simulink model "sm_parts_all"  (R2019a)
settings: Solver=VariableStepAuto  StartTime=0.0  StopTime=10.0  RelTol=1e-3  EnableMultiTasking=on
undefined symbols (not defined in the file): X, Y, Z
libraries: sm_lib x19, Multibody_Parts_Lib x18, nesl_utility x1
Description:
  | Copyright 2017-2019 The MathWorks, Inc.
settings Model: Creator=smiller  LastModifiedBy=smiller
settings DataIOCC: LimitDataPoints=on  ReturnWorkspaceOutputs=off
settings OptimizationCC: LifeSpan=inf
settings DebuggingCC: AllowSymbolicDim=off  PregeneratedLibrarySubsystemCodeDiagnostic=none  SFUnexpectedBacktrackingDiag=warning  SFNoUnconditionalDefaultTransitionDiag=warning  SFExecutionAtInitializationDiag=none  ArithmeticOperatorsInVariantConditions=warning
settings SFSimCC: SimUseLocalCustomCode=off
settings RTWCC: RTWUseLocalCustomCode=off
settings CodeAppCC: StateflowObjectComments=on
settings GRTTargetCC: TargetLangStandard=C89/C90 (ANSI)  GeneratePreprocessorConditionals=Disable all
settings ConfigComp: CovMetricSettings=dw  CovHtmlReporting=on  CovSaveCumulativeToWorkspaceVar=on  CovSaveSingleToWorkspaceVar=on  CovExternalEMLEnable=off  CovSFcnEnable=off
settings SimscapeCC: SimscapeNormalizeSystem=off  SimscapeLogType=all  SimscapeLogDataHistory=10000
settings ConfigurationSet: Description=SimMechanics 2G
settings ExplorerConfigSet: InternalSimMechanicsExplorerSettings="<ExplorerConfiguration><canonicalview>default</canonicalview><AnimationSetting><BasePlaybackSpeed>1.0</BasePlaybackSpeed><PlaybackSpeedFactor>1.0</PlaybackSpeedFactor></AnimationSetting><TilePanel><TileInfo><Tiles Columns=\"1\" Count=\"1\" Rows=\"1\"><Column Left=\"2\" Weight=\"1\"/><Column Left=\"401\"/><Row Top=\"2\" Weight=\"1\"/><Row Top=\"205\"/><Tile Height=\"1\" Width=\"1\" X=\"0\" Y=\"0\"/></Tiles></TileInfo><SceneInfo><SceneViewer><BGColor><R>1</R><G>1</G><B>1</B></BGColor><Camera><DoPerspective>off</DoPerspective><Position><X>-0.71015375614700837</X><Y>0.14184611226395488</Y><Z>-0.013997968745046566</Z></Position><Center><X>0.28084060208517991</X><Y>0.025638016485088261</Y><Z>-0.080525109277487794</Z></Center><Up><X>0.11482264391220898</X><Y>0.99308884035982059</Y><Z>-0.024296411212304969</Z></Up><ViewLimDist>1</ViewLimDist><YLim>0.095367858286087334</YLim><XLim>0.19171889036893844</XLim></Camera></SceneViewer></SceneInfo></TilePanel><MechEditorPanel><Cameras/><GfxPanelCameraMap/><VideoCreator><PlaybackSpeedRatio>1.0</PlaybackSpeedRatio><FrameRate>30</FrameRate><VideoFormat>Motion JPEG AVI</VideoFormat><FrameSize>auto</FrameSize></VideoCreator></MechEditorPanel></ExplorerConfiguration>"

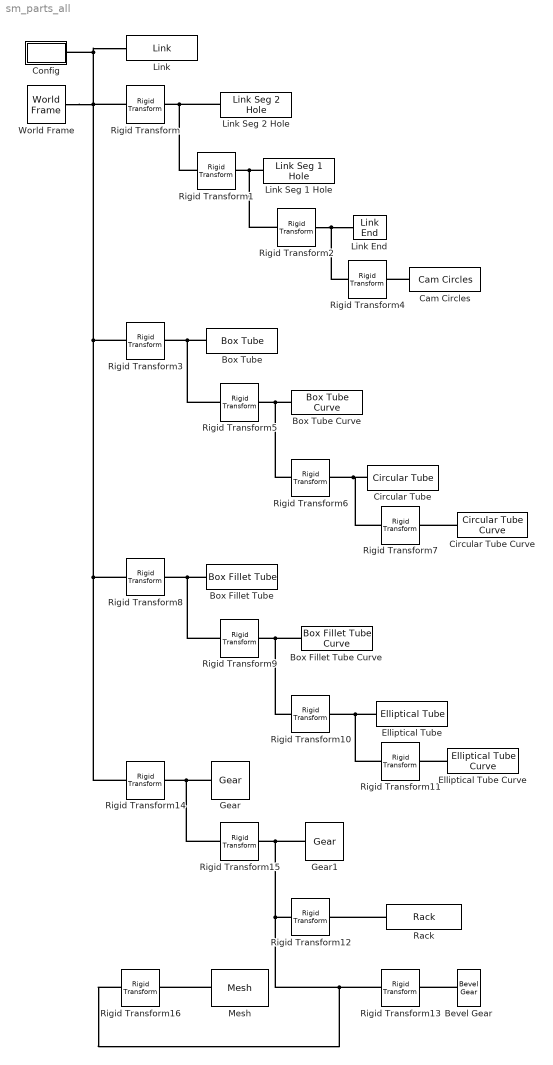
== system sm_parts_all ==
  Bevel Gear : Multibody_Parts_Lib/Gears/Bevel Gear  gear_ra=0.03  gear_th=0.01  gear_ca=90/2  gear_hr=0.002  gear_rho=7000  gear_clr=[0.0 0.4 0.6]  gear_opc=1  popup_markings=Two  mark_radius_range=[0.7 0.8]  mark_angle_range=60  mark_color=[1 1 1]
      settings: SourceProductName=Simscape Multibody Parts Library
  Box Fillet Tube : Multibody_Parts_Lib/Extrusions/Box Fillet Tube  box_ox=0.02  box_ix=0.01  box_oy=0.028  box_iy=0.018  rad_o=0.005  rad_i=0.002  box_len=0.05  box_rho=7000  box_color=[0 0.4 0.6]  box_opc=1
      settings: SourceProductName=Simscape Multibody Parts Library
  Box Fillet Tube Curve : Multibody_Parts_Lib/Extrusions/Box Fillet Tube Curve  box_ox=0.02  box_ix=0.01  box_oy=0.028  box_iy=0.018  rad_o=0.005  rad_i=0.002  arc_rad=0.05  arc_angle=45  popup_arcdir=Z  box_rho=7000  box_color=[0 0.4 0.6]  box_opc=1
      settings: SourceProductName=Simscape Multibody Parts Library
  Box Tube : Multibody_Parts_Lib/Extrusions/Box Tube  box_ox=0.02  box_ix=0.01  box_oy=0.028  box_iy=0.018  box_len=0.05  box_rho=7000  box_color=[0 0.4 0.6]  box_opc=1
      settings: SourceProductName=Simscape Multibody Parts Library
  Box Tube Curve : Multibody_Parts_Lib/Extrusions/Box Tube Curve  box_ox=0.02  box_ix=0.01  box_oy=0.028  box_iy=0.018  arc_rad=0.05  arc_angle=45  popup_arcdir=Z  box_rho=7000  box_color=[0 0.4 0.6]  box_opc=1
      settings: SourceProductName=Simscape Multibody Parts Library
  Cam Circles : Multibody_Parts_Lib/Linkages/Cam Circles  rad_b=0.02  rad_f=0.01  radhb=0.005  radhf=0.005  cam_len=0.05  cam_thickness=0.01  cam_rho=7000  cam_color=[0 0.4 0.6]  cam_opc=1
      settings: SourceProductName=Simscape Multibody Parts Library
  Circular Tube : Multibody_Parts_Lib/Extrusions/Circular Tube  circ_radout=0.015  circ_radin=0.01  deg_1=45  deg_2=315  circ_len=0.05  circ_rho=7000  circ_color=[0 0.4 0.6]  circ_opc=1
      settings: SourceProductName=Simscape Multibody Parts Library
  Circular Tube Curve : Multibody_Parts_Lib/Extrusions/Circular Tube Curve  circ_radout=0.015  circ_radin=0.01  deg_1=45  deg_2=315  arc_rad=0.05  arc_angle=45  popup_arcdir=Z  circ_rho=7000  circ_color=[0 0.4 0.6]  circ_opc=1
      settings: SourceProductName=Simscape Multibody Parts Library
  Config : Subsystem
  Elliptical Tube : Multibody_Parts_Lib/Extrusions/Elliptical Tube  rad_a=0.006  rad_b=0.015  deg_1=10  deg_2=350  ctr=0.7  ell_len=0.05  ell_rho=7000  ell_color=[0 0.4 0.6]  ell_opc=1
      settings: SourceProductName=Simscape Multibody Parts Library
  Elliptical Tube Curve : Multibody_Parts_Lib/Extrusions/Elliptical Tube Curve  rad_a=0.006  rad_b=0.015  deg_1=10  deg_2=350  ctr=0.7  arc_rad=0.05  arc_angle=45  popup_arcdir=Z  ell_rho=7000  ell_color=[0 0.4 0.6]  ell_opc=1
      settings: SourceProductName=Simscape Multibody Parts Library
  Gear : Multibody_Parts_Lib/Gears/Gear  popup_gear_type=External  gear_pd=0.035  gear_nt=12  gear_th=0.02  gear_rh=0.005  gear_rt=0.02  gear_rho=7000  gear_clr=[0.0 0.4 0.6]  gear_opc=1  popup_ad_dd=Default  gear_ad=0.125/12  gear_dd=1.157*0.125/12  popup_markings=Two  mark_radius_range=[0.6 0.7]  mark_angle_range=60  mark_color=[1 1 1]
      settings: SourceProductName=Simscape Multibody Parts Library
  Gear1 : Multibody_Parts_Lib/Gears/Gear  popup_gear_type=Internal  gear_pd=0.035  gear_nt=12  gear_th=0.02  gear_rh=0.005  gear_rt=0.002  gear_rho=7000  gear_clr=[0.0 0.4 0.6]  gear_opc=1  popup_ad_dd=Default  gear_ad=0.125/12  gear_dd=1.157*0.125/12  popup_markings=Two  mark_radius_range=[1.23 1.28]  mark_angle_range=60  mark_color=[1 1 1]
      settings: SourceProductName=Simscape Multibody Parts Library
  Link : Multibody_Parts_Lib/Linkages/Link  link_len=0.05  link_width=0.025  link_radh=0.005  link_numh=3  link_thickness=0.01  link_rho=7000  link_color=[0 0.4 0.6]  link_opc=1
      settings: SourceProductName=Simscape Multibody Parts Library
  Link End : Multibody_Parts_Lib/Linkages/Link End  circ_radout=0.025/2  circ_radin=0.005  popup_holelr=+X  deg_1=-90  deg_2=90  circ_len=0.01  circ_rho=7000  circ_color=[0 0.4 0.6]  circ_opc=1
      settings: SourceProductName=Simscape Multibody Parts Library
  Link Seg 1 Hole : Multibody_Parts_Lib/Linkages/Link Seg 1 Hole  link_len=0.05  link_width=0.025  link_radh=0.005  link_holelr=+X  link_thickness=0.01  link_rho=7000  link_color=[0 0.4 0.6]  link_opc=1
      settings: SourceProductName=Simscape Multibody Parts Library
  Link Seg 2 Hole : Multibody_Parts_Lib/Linkages/Link Seg 2 Hole  link_len=0.05  link_width=0.025  link_radh=0.005  link_thickness=0.01  link_rho=7000  link_color=[0 0.4 0.6]  link_opc=1
      settings: SourceProductName=Simscape Multibody Parts Library
  Mesh : Multibody_Parts_Lib/Basic/Mesh  mesh_lenx=0.06  mesh_leny=0.03  mesh_hx=0.0045  mesh_hy=0.0045  mesh_numhx=6  mesh_numhy=3  mesh_thickness=0.02  mesh_rho=7000  mesh_color=[0 0.4 0.6]  mesh_opc=1
      settings: SourceProductName=Simscape Multibody Parts Library
  Rack : Multibody_Parts_Lib/Gears/Rack  rack_tp=0.01  rack_nt=5  rack_tb=0.006  rack_th=0.006  rack_rho=7000  rack_clr=[0.5 0.5 0.5]  rack_opc=1  popup_ad_dd=Default  rack_ad=0.052/pi  rack_dd=1.157*0.052/pi
      settings: SourceProductName=Simscape Multibody Parts Library
  Rigid Transform{,1..2,4} (4 alike) : sm_lib/Frames and Transforms/Rigid Transform  TranslationMethod=StandardAxis  TranslationStandardOffset=0.05  TranslationLengthUnit=m  TranslationStandardAxis=+Y  TranslationCartesianOffset=[0 0 0]  TranslationROffset=0  TranslationROffsetUnits=m  TranslationZOffset=0  TranslationZOffsetUnits=m  TranslationThetaOffset=0  TranslationThetaOffsetUnits=deg  RotationMethod=None  RotationAngleUnits=deg  RotationStandardAxis=+Z  RotationAngle=0.0  RotationArbitraryAxis=[0 0 1]  FollAlignAxisA=+X  BaseAlignAxisA=+Y  FollAlignAxisB=+Y  BaseAlignAxisB=+Z  RotationSequenceAxes=FollowerAxes  RotationSequence=XYX  RotationSequenceAngles=[0 0 0]  RotationSequenceAnglesUnits=deg  RotationMatrix=[1 0 0; 0 1 0; 0 0 1]
  Rigid Transform{5..7,9..11,15} (7 alike) : sm_lib/Frames and Transforms/Rigid Transform  TranslationMethod=StandardAxis  TranslationStandardOffset=0.05  TranslationLengthUnit=m  TranslationStandardAxis=+Y  TranslationCartesianOffset=[0 0 0]  TranslationROffset=0  TranslationROffsetUnits=m  TranslationZOffset=0  TranslationZOffsetUnits=m  TranslationThetaOffset=0  TranslationThetaOffsetUnits=deg  RotationMethod=None  RotationAngleUnits=deg  RotationStandardAxis=+Y  RotationAngle=0  RotationArbitraryAxis=[0 0 1]  FollAlignAxisA=+X  BaseAlignAxisA=+Y  FollAlignAxisB=+Y  BaseAlignAxisB=+Z  RotationSequenceAxes=FollowerAxes  RotationSequence=XYX  RotationSequenceAngles=[0 0 0]  RotationSequenceAnglesUnits=deg  RotationMatrix=[1 0 0; 0 1 0; 0 0 1]
  Rigid Transform12 : sm_lib/Frames and Transforms/Rigid Transform  TranslationMethod=StandardAxis  TranslationStandardOffset=0.05  TranslationLengthUnit=m  TranslationStandardAxis=+Y  TranslationCartesianOffset=[0 0 0]  TranslationROffset=0  TranslationROffsetUnits=m  TranslationZOffset=0  TranslationZOffsetUnits=m  TranslationThetaOffset=0  TranslationThetaOffsetUnits=deg  RotationMethod=AlignedAxes  RotationAngleUnits=deg  RotationStandardAxis=+Y  RotationAngle=0  RotationArbitraryAxis=[0 0 1]  FollAlignAxisA=+Z  BaseAlignAxisA=+Y  FollAlignAxisB=+Y  BaseAlignAxisB=+X  RotationSequenceAxes=FollowerAxes  RotationSequence=XYX  RotationSequenceAngles=[0 0 0]  RotationSequenceAnglesUnits=deg  RotationMatrix=[1 0 0; 0 1 0; 0 0 1]
  Rigid Transform13 : sm_lib/Frames and Transforms/Rigid Transform  TranslationMethod=StandardAxis  TranslationStandardOffset=0.1  TranslationLengthUnit=m  TranslationStandardAxis=+Y  TranslationCartesianOffset=[0 0 0]  TranslationROffset=0  TranslationROffsetUnits=m  TranslationZOffset=0  TranslationZOffsetUnits=m  TranslationThetaOffset=0  TranslationThetaOffsetUnits=deg  RotationMethod=StandardAxis  RotationAngleUnits=deg  RotationStandardAxis=+X  RotationAngle=-75  RotationArbitraryAxis=[0 0 1]  FollAlignAxisA=+X  BaseAlignAxisA=+Y  FollAlignAxisB=+Y  BaseAlignAxisB=+Z  RotationSequenceAxes=FollowerAxes  RotationSequence=XYX  RotationSequenceAngles=[0 0 0]  RotationSequenceAnglesUnits=deg  RotationMatrix=[1 0 0; 0 1 0; 0 0 1]
  Rigid Transform14 : sm_lib/Frames and Transforms/Rigid Transform  TranslationMethod=StandardAxis  TranslationStandardOffset=0.15  TranslationLengthUnit=m  TranslationStandardAxis=-X  TranslationCartesianOffset=[0 0 0]  TranslationROffset=0  TranslationROffsetUnits=m  TranslationZOffset=0  TranslationZOffsetUnits=m  TranslationThetaOffset=0  TranslationThetaOffsetUnits=deg  RotationMethod=StandardAxis  RotationAngleUnits=deg  RotationStandardAxis=+Y  RotationAngle=0  RotationArbitraryAxis=[0 0 1]  FollAlignAxisA=+X  BaseAlignAxisA=+Y  FollAlignAxisB=+Y  BaseAlignAxisB=+Z  RotationSequenceAxes=FollowerAxes  RotationSequence=XYX  RotationSequenceAngles=[0 0 0]  RotationSequenceAnglesUnits=deg  RotationMatrix=[1 0 0; 0 1 0; 0 0 1]
  Rigid Transform16 : sm_lib/Frames and Transforms/Rigid Transform  TranslationMethod=StandardAxis  TranslationStandardOffset=0.15  TranslationLengthUnit=m  TranslationStandardAxis=+Y  TranslationCartesianOffset=[-0.2 0.05 0]  TranslationROffset=0  TranslationROffsetUnits=m  TranslationZOffset=0  TranslationZOffsetUnits=m  TranslationThetaOffset=0  TranslationThetaOffsetUnits=deg  RotationMethod=StandardAxis  RotationAngleUnits=deg  RotationStandardAxis=+Y  RotationAngle=0  RotationArbitraryAxis=[0 0 1]  FollAlignAxisA=+X  BaseAlignAxisA=+Y  FollAlignAxisB=+Y  BaseAlignAxisB=+Z  RotationSequenceAxes=FollowerAxes  RotationSequence=XYX  RotationSequenceAngles=[0 0 0]  RotationSequenceAnglesUnits=deg  RotationMatrix=[1 0 0; 0 1 0; 0 0 1]
  Rigid Transform3 : sm_lib/Frames and Transforms/Rigid Transform  TranslationMethod=StandardAxis  TranslationStandardOffset=0.05  TranslationLengthUnit=m  TranslationStandardAxis=-X  TranslationCartesianOffset=[0 0 0]  TranslationROffset=0  TranslationROffsetUnits=m  TranslationZOffset=0  TranslationZOffsetUnits=m  TranslationThetaOffset=0  TranslationThetaOffsetUnits=deg  RotationMethod=StandardAxis  RotationAngleUnits=deg  RotationStandardAxis=+Y  RotationAngle=80  RotationArbitraryAxis=[0 0 1]  FollAlignAxisA=+X  BaseAlignAxisA=+Y  FollAlignAxisB=+Y  BaseAlignAxisB=+Z  RotationSequenceAxes=FollowerAxes  RotationSequence=XYX  RotationSequenceAngles=[0 0 0]  RotationSequenceAnglesUnits=deg  RotationMatrix=[1 0 0; 0 1 0; 0 0 1]
  Rigid Transform8 : sm_lib/Frames and Transforms/Rigid Transform  TranslationMethod=StandardAxis  TranslationStandardOffset=0.1  TranslationLengthUnit=m  TranslationStandardAxis=-X  TranslationCartesianOffset=[0 0 0]  TranslationROffset=0  TranslationROffsetUnits=m  TranslationZOffset=0  TranslationZOffsetUnits=m  TranslationThetaOffset=0  TranslationThetaOffsetUnits=deg  RotationMethod=StandardAxis  RotationAngleUnits=deg  RotationStandardAxis=+Y  RotationAngle=80  RotationArbitraryAxis=[0 0 1]  FollAlignAxisA=+X  BaseAlignAxisA=+Y  FollAlignAxisB=+Y  BaseAlignAxisB=+Z  RotationSequenceAxes=FollowerAxes  RotationSequence=XYX  RotationSequenceAngles=[0 0 0]  RotationSequenceAnglesUnits=deg  RotationMatrix=[1 0 0; 0 1 0; 0 0 1]
  World Frame : sm_lib/Frames and Transforms/World Frame
  connections:
  World Frame/RConn1 -- Rigid Transform14/LConn1 -- Rigid Transform8/LConn1 -- Rigid Transform3/LConn1 -- Link/LConn1 -- Config/LConn1 -- Rigid Transform/LConn1
  Link Seg 2 Hole/LConn1 -- Rigid Transform1/LConn1 -- Rigid Transform/RConn1
  Link Seg 1 Hole/LConn1 -- Rigid Transform2/LConn1 -- Rigid Transform1/RConn1
  Rigid Transform2/RConn1 -- Rigid Transform4/LConn1 -- Link End/LConn1
  Box Tube/LConn1 -- Rigid Transform5/LConn1 -- Rigid Transform3/RConn1
  Cam Circles/LConn1 -- Rigid Transform4/RConn1
  Box Tube Curve/LConn1 -- Rigid Transform6/LConn1 -- Rigid Transform5/RConn1
  Circular Tube/LConn1 -- Rigid Transform7/LConn1 -- Rigid Transform6/RConn1
  Circular Tube Curve/LConn1 -- Rigid Transform7/RConn1
  Rigid Transform9/LConn1 -- Box Fillet Tube/LConn1 -- Rigid Transform8/RConn1
  Rigid Transform10/LConn1 -- Box Fillet Tube Curve/LConn1 -- Rigid Transform9/RConn1
  Rigid Transform11/LConn1 -- Elliptical Tube/LConn1 -- Rigid Transform10/RConn1
  Elliptical Tube Curve/LConn1 -- Rigid Transform11/RConn1
  Rigid Transform15/RConn1 -- Rigid Transform16/LConn1 -- Rigid Transform13/LConn1 -- Rigid Transform12/LConn1 -- Gear1/RConn1
  Rack/RConn1 -- Rigid Transform12/RConn1
  Bevel Gear/RConn1 -- Rigid Transform13/RConn1
  Rigid Transform14/RConn1 -- Gear/RConn1 -- Rigid Transform15/LConn1
  Mesh/LConn1 -- Rigid Transform16/RConn1

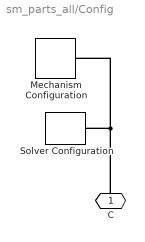
== system sm_parts_all/Config ==
  Mechanism Configuration : sm_lib/Utilities/Mechanism Configuration  UniformGravity=Constant  GravityVector=[0 0 -9.80665]  GravityUnits=m/s^2  LinearizationDelta=0.001
  Solver Configuration : nesl_utility/Solver Configuration  PhysicalDomain=network_engine_domain  SubClassName=solver  LeftPortType=input  RightPortType=generic  Tones=[]  Harmonics=[]  SimulateNoise=off  Profile=off  UseLocalSampling=off  EnableSwitchedLinearOptims=on  FrequencyDomain=off  UseCCode=off  RelTol=0.001  AbsTol=1e-06  MinStep=1e-09  ToWorkspace=off  RevertToSquareIcSolve=off  NumHomotopyIterations=100  PhasorMode=off  PhasorModeNumHarmonics=1  DoDC=off  ResidualTolerance=1e-09  UseLocalSolver=off  LocalSolverChoice=NE_BACKWARD_EULER_ADVANCER  LocalSolverSampleTime=0.001  DoFixedCost=off  MaxNonlinIter=3  MaxModeIter=2  LinearAlgebra=Sparse  EquationFormulation=NE_TIME_EF  DelaysMemoryBudget=1024  AutomaticFiltering=on  FilteringTimeConstant=0.001  PartitionStorageMethod=AS_NEEDED  PartitionMemoryBudget=1024  PartitionMethod=FAST
  C : PMIOPort  Side=Left
  connections:
  Mechanism Configuration/RConn1 -- C/RConn1 -- Solver Configuration/RConn1
